simulink model "test_horizon2body"  (R2015b)
settings: Solver=FixedStepAuto  StartTime=0.0  StopTime=10  FixedStep=0.1  RelTol=1e-3
libraries: simulink_extras x2
settings Model: Creator=rcasado  LastModifiedBy=rcasado

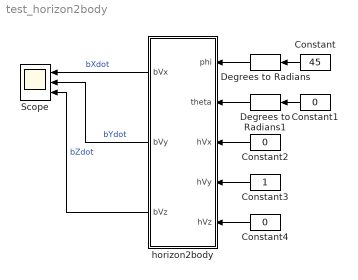
== system test_horizon2body ==
  Constant : Constant  Value=45
  Constant1 : Constant  Value=0
  Constant2 : Constant  Value=0
  Constant3 : Constant
  Constant4 : Constant  Value=0
  Degrees to Radians : simulink_extras/Transformations/Degrees to Radians
  Degrees to Radians1 : simulink_extras/Transformations/Degrees to Radians
  Scope : Scope  NumInputPorts=3
  horizon2body : Subsystem
  wires:
  horizon2body/3(bVz) -> Scope/3  "bZdot"
  horizon2body/1(bVx) -> Scope/1  "bXdot"
  horizon2body/2(bVy) -> Scope/2  "bYdot"
  Constant/1 -> Degrees to Radians/1
  Degrees to Radians/1 -> horizon2body/1(phi)
  Constant1/1 -> Degrees to Radians1/1
  Degrees to Radians1/1 -> horizon2body/2(theta)
  Constant4/1 -> horizon2body/5(hVz)
  Constant3/1 -> horizon2body/4(hVy)
  Constant2/1 -> horizon2body/3(hVx)

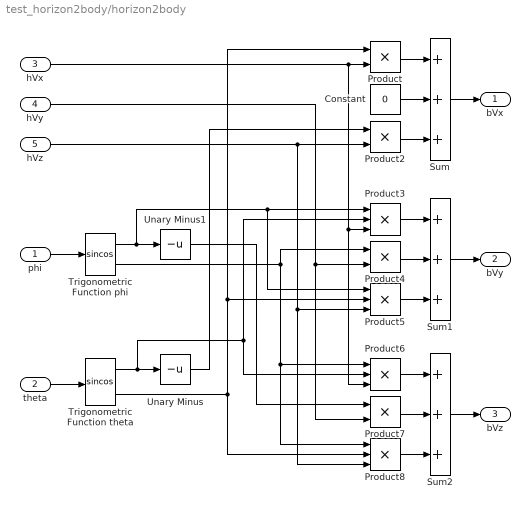
== system test_horizon2body/horizon2body ==
  phi : Inport
  theta : Inport  Port=2
  hVx : Inport  Port=3
  hVy : Inport  Port=4
  hVz : Inport  Port=5
  Constant : Constant  Value=0
  Product{,2,4,7} (4 alike) : Product
  Product{3,5..6,8} (4 alike) : Product  Inputs=3
  Sum : Sum  Inputs=3
  Sum1 : Sum  Inputs=3
  Sum2 : Sum  Inputs=3
  Trigonometric Function phi : Trigonometry  Operator=sincos
  Trigonometric Function theta : Trigonometry  Operator=sincos
  Unary Minus : UnaryMinus
  Unary Minus1 : UnaryMinus
  bVx : Outport
  bVy : Outport  Port=2
  bVz : Outport  Port=3
  wires:
  theta/1 -> Trigonometric Function theta/1
  phi/1 -> Trigonometric Function phi/1
  Trigonometric Function phi/2 -> Product4/1, Product8/1, Product6/1
  Trigonometric Function theta/2 -> Product8/2, Product/1, Product5/2
  Trigonometric Function theta/1 -> Product3/2, Product6/2, Unary Minus/1
  Trigonometric Function phi/1 -> Unary Minus1/1, Product5/1, Product3/1
  Sum/1 -> bVx/1
  Sum1/1 -> bVy/1
  Sum2/1 -> bVz/1
  Product/1 -> Sum/1
  Constant/1 -> Sum/2
  Product2/1 -> Sum/3
  Product3/1 -> Sum1/1
  Product4/1 -> Sum1/2
  Product5/1 -> Sum1/3
  Product6/1 -> Sum2/1
  Product7/1 -> Sum2/2
  Product8/1 -> Sum2/3
  hVx/1 -> Product6/3, Product3/3, Product/2
  hVy/1 -> Product7/2, Product4/2
  hVz/1 -> Product8/3, Product5/3, Product2/2
  Unary Minus/1 -> Product2/1
  Unary Minus1/1 -> Product7/1
